simulink model "SineSystem"  (R2020a)
settings: Solver=VariableStepAuto  StartTime=0.0  StopTime=10.0  RelTol=1e-3
settings Model: Creator=jiaweichen  LastModifiedBy=jiaweichen
settings DataIOCC: SaveFormat=Array

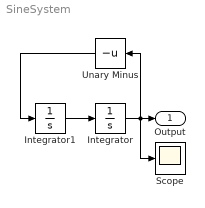
== system SineSystem ==
  Integrator : Integrator
  Integrator1 : Integrator  InitialCondition=1
  Scope : Scope
  Unary Minus : UnaryMinus
  Output : Outport
  wires:
  Integrator/1 -> Scope/1, Output/1, Unary Minus/1
  Integrator1/1 -> Integrator/1
  Unary Minus/1 -> Integrator1/1
